simulink model "com_test"  (R2021b)
settings: Solver=VariableStepAuto  StartTime=0.0  StopTime=10.0  RelTol=1e-3
libraries: slrealtimeseriallib x2, instrumentlib x2, slrealtimeutilitieslib x1, etargetslib x1
settings Model: Creator=riku3  LastModifiedBy=riku3

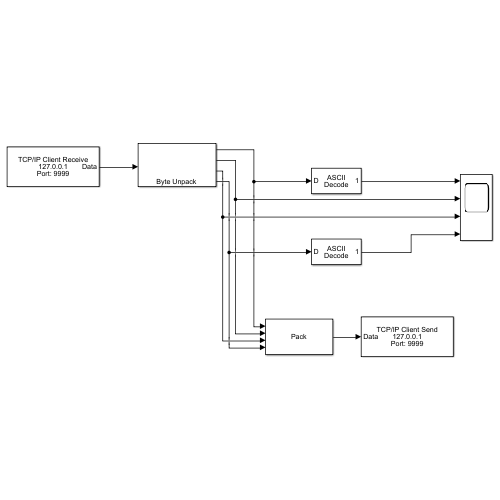
[thumbnail: Simulink's stored preview of the top-level diagram]
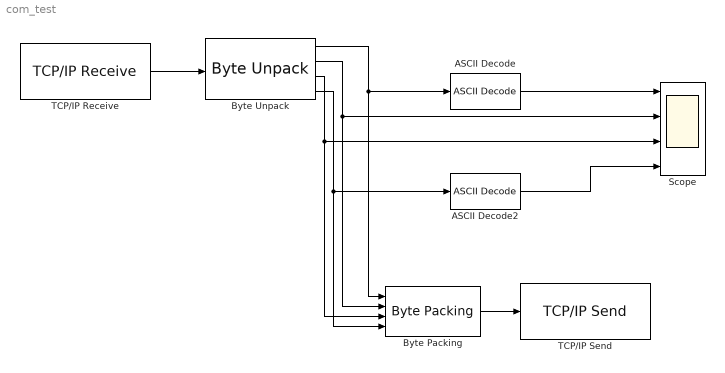
== system com_test ==
  ASCII Decode : slrealtimeseriallib/ASCII Decode  format=%d\r  nvars=1  vartypes={ }
      settings: SourceProductBaseCode=XP
  ASCII Decode2 : slrealtimeseriallib/ASCII Decode  format=%d\r  nvars=1  vartypes={ }
      settings: SourceProductBaseCode=XP
  Byte Packing : slrealtimeutilitieslib/Byte Packing  MaskPackedDataType=uint8  MaskUnpackedDataTypes={'uint8','uint8','uint8','uint8'}  MaskAlignment=2
  Byte Unpack : etargetslib/Byte Unpack  dimensions={[1],[1],[1],[1]}  datatypes={'uint8','uint8','uint8','uint8'}  byteAlign=1
  Scope : Scope  NumInputPorts=4
  TCP/IP Receive : instrumentlib/TCP//IP Receive  Host=127.0.0.1  Port=9999  DataSize=[4]  DataType=uint8  ASCIIFormatting=%d  Terminator=LF  CustomTerminator=10  ByteOrder=big-endian  EnableBlockingMode=on  Timeout=10  SampleTime=0.1  SimulateUsing=Interpreted execution
  TCP/IP Send : instrumentlib/TCP//IP Send  Host=127.0.0.1  Port=9999  ByteOrder=big-endian  EnableBlockingMode=on  Timeout=10  TransferDelay=on  SimulateUsing=Interpreted execution
  wires:
  Byte Unpack/1 -> ASCII Decode/1, Byte Packing/1
  Byte Packing/1 -> TCP/IP Send/1
  TCP/IP Receive/1 -> Byte Unpack/1
  Byte Unpack/4 -> ASCII Decode2/1, Byte Packing/4
  Byte Unpack/2 -> Byte Packing/2, Scope/2
  ASCII Decode/1 -> Scope/1
  Byte Unpack/3 -> Scope/3, Byte Packing/3
  ASCII Decode2/1 -> Scope/4
